simulink model "EXPERIMENT_03"  (R2023b)
settings: Solver=VariableStepAuto  StartTime=0.0  StopTime=0.2  RelTol=1e-3
libraries: spsRMSLib x24, spsPowerLib x16, spsVoltageMeasurementLib x16, spsSeriesRLCBranchLib x15, spsACVoltageSourceLib x8, spsCurrentMeasurementLib x8, spsSeriesRLCLoadLib x8, sps_lib x1
settings Model: Creator=deves  LastModifiedBy=deves

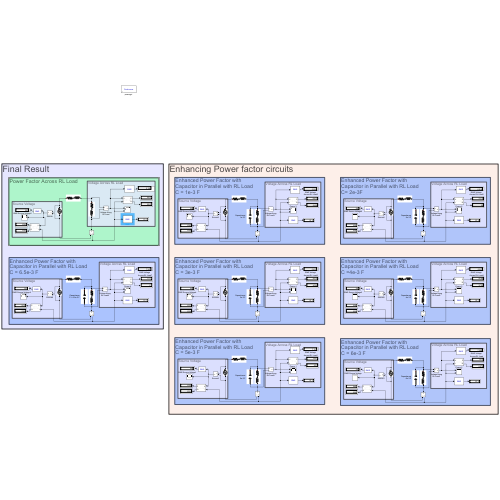
[thumbnail: Simulink's stored preview of the top-level diagram]
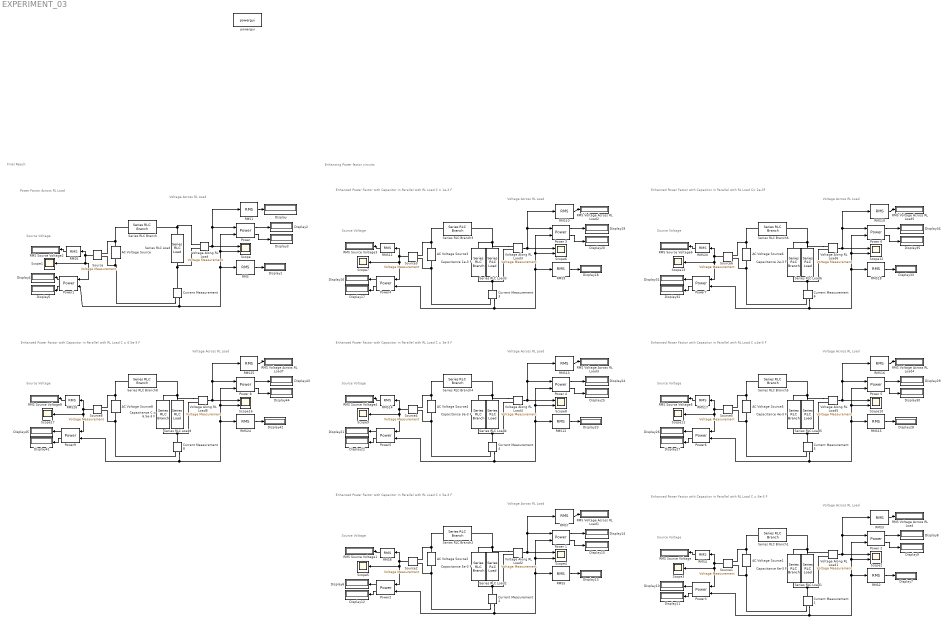
== system EXPERIMENT_03 ==
  note: Final Result
  note: Enhancing Power factor circuits
  note: Enhanced Power Factor with
      | Capacitor in Parallel with RL Load
      | C = 6e-3 F
  note: Power Factor Across RL Load
  note: Source Voltage
  note: Voltage Across RL Load
  note: Voltage Across RL Load
  note: Source Voltage
  note: Voltage Across RL Load
  note: Source Voltage
  note: Enhanced Power Factor with
      | Capacitor in Parallel with RL Load
      | C = 5e-3 F
  note: Voltage Across RL Load
  note: Source Voltage
  note: Enhanced Power Factor with
      | Capacitor in Parallel with RL Load
      | C = 1e-3 F
  note: Voltage Across RL Load
  note: Source Voltage
  note: Enhanced Power Factor with
      | Capacitor in Parallel with RL Load
      | C = 3e-3 F
  note: Voltage Across RL Load
  note: Source Voltage
  note: Enhanced Power Factor with
      | Capacitor in Parallel with RL Load
      | C =4e-3 F
  note: Voltage Across RL Load
  note: Source Voltage
  note: Enhanced Power Factor with
      | Capacitor in Parallel with RL Load
      | C= 2e-3F
  note: Enhanced Power Factor with
      | Capacitor in Parallel with RL Load
      | C = 6.5e-3 F
  note: Voltage Across RL Load
  note: Source Voltage
  AC Voltage Source{,1..6,8} (8 alike) : spsACVoltageSourceLib/AC Voltage Source  Amplitude=220*sqrt(2)  Phase=0  Frequency=50  SampleTime=.0001  Measurements=None  BusType=swing  Pref=10e3  Qref=0  Qmin=-inf  Qmax=+inf
  Capacitance 1e-3 F : spsSeriesRLCBranchLib/Series RLC Branch  LConnTagsString=__new0  RConnTagsString=__new0  BranchType=C  Resistance=1  Inductance=1e-3  SetiL0=off  InitialCurrent=0  Capacitance=1e-3  Setx0=off  InitialVoltage=0  Measurements=None
  Capacitance 2e-3 F : spsSeriesRLCBranchLib/Series RLC Branch  LConnTagsString=__new0  RConnTagsString=__new0  BranchType=C  Resistance=1  Inductance=1e-3  SetiL0=off  InitialCurrent=0  Capacitance=2e-3  Setx0=off  InitialVoltage=0  Measurements=None
  Capacitance 3e-3 F : spsSeriesRLCBranchLib/Series RLC Branch  LConnTagsString=__new0  RConnTagsString=__new0  BranchType=C  Resistance=1  Inductance=1e-3  SetiL0=off  InitialCurrent=0  Capacitance=3e-3  Setx0=off  InitialVoltage=0  Measurements=None
  Capacitance 4e-3 F : spsSeriesRLCBranchLib/Series RLC Branch  LConnTagsString=__new0  RConnTagsString=__new0  BranchType=C  Resistance=1  Inductance=1e-3  SetiL0=off  InitialCurrent=0  Capacitance=4e-3  Setx0=off  InitialVoltage=0  Measurements=None
  Capacitance 5e-3 F : spsSeriesRLCBranchLib/Series RLC Branch  LConnTagsString=__new0  RConnTagsString=__new0  BranchType=C  Resistance=1  Inductance=1e-3  SetiL0=off  InitialCurrent=0  Capacitance=5e-3  Setx0=off  InitialVoltage=0  Measurements=None
  Capacitance 6e-3 F : spsSeriesRLCBranchLib/Series RLC Branch  LConnTagsString=__new0  RConnTagsString=__new0  BranchType=C  Resistance=1  Inductance=1e-3  SetiL0=off  InitialCurrent=0  Capacitance=6e-3  Setx0=off  InitialVoltage=0  Measurements=None
  Capacitance C = 6.5e-3 F : spsSeriesRLCBranchLib/Series RLC Branch  LConnTagsString=__new0  RConnTagsString=__new0  BranchType=C  Resistance=1  Inductance=1e-3  SetiL0=off  InitialCurrent=0  Capacitance=6.5e-3  Setx0=off  InitialVoltage=0  Measurements=None
  Current Measurement{,1..6,8} (8 alike) : spsCurrentMeasurementLib/Current Measurement  PhasorSimulation=off  OutputType=Complex  PSBequivalent=0
  Display{,1..35,41..45} (41 alike) : Display
  Power{,1..7,9} (9 alike) : spsPowerLib/Power  Freq=50  Vinit=[1, 0]  Iinit=[1, 0]  Ts=0
  Power {1..6,8} (7 alike) : spsPowerLib/Power  Freq=50  Vinit=[1, 0]  Iinit=[1, 0]  Ts=0
  RMS{,1..20,24..26} (24 alike) : spsRMSLib/RMS  TrueRMS=on  Freq=50  RMSInit=120  Ts=0
  RMS Source Voltage{,1..6,8} (8 alike) : Display
  RMS Voltage Across RL Load{,1..5,7} (7 alike) : Display
  Scope{,2,4,6,8,10,12,16} (8 alike) : Scope  NumInputPorts=2
  Scope{1,3,5,7,9,11,13,17} (8 alike) : Scope
  Series RLC Branch{,1..6,8} (8 alike) : spsSeriesRLCBranchLib/Series RLC Branch  LConnTagsString=__new0  RConnTagsString=__new0  BranchType=RL  Resistance=10  Inductance=3.183e-2  SetiL0=off  InitialCurrent=0  Capacitance=1e-6  Setx0=off  InitialVoltage=0  Measurements=None
  Series RLC Load{,1..6,8} (8 alike) : spsSeriesRLCLoadLib/Series RLC Load  LConnTagsString=a  RConnTagsString=__new0  NominalVoltage=220  NominalFrequency=50  ActivePower=10e4  InductivePower=10e4  CapacitivePower=0  Setx0=off  InitialVoltage=0  SetiL0=off  InitialCurrent=0  Measurements=None  LoadType=constant Z
  Source{,1..6,8} (8 alike) : spsVoltageMeasurementLib/Voltage Measurement  PhasorSimulation=off  OutputType=Complex  PSBequivalent=0
  Voltage Along RL Load{,1..6,8} (8 alike) : spsVoltageMeasurementLib/Voltage Measurement  PhasorSimulation=off  OutputType=Complex  PSBequivalent=0
  powergui : sps_lib/powergui  Priority=1  SimulationMode=Continuous  SampleTime=50e-6  frequency=60  Iterations=50  frequencyindice=50  Pbase=100e6  ErrMax=1e-4  UnitsV=kV  UnitsW=MW  buscounter=0  FunctionMessages=off  echomessages=off  EnableUseOfTLC=off  CurrentSourceSwitches=off  DisableSnubberDevices=off  DisableRonSwitches=off  DisableVfSwitches=off  DisplayEquations=off  AutomaticDiscreteSolvers=off  SolverType=Tustin/Backward Euler (TBE)  Interpol=off  ExternalGateDelay=off  methode=off  Ts=100  x0status=blocks  SPID=on  SwTol=0  HookPort=off  NonlinearTolerance=1e-4  nMaxIteration=100  ContinueOnMaxIteration=off  RestoreLinks=warning  ResistiveCurrentMeasurement=off  Frange=[0:2:500]  Ylog=off  Xlog=on  ShowGrid=off  save=off  variable=ZData  structure=0  ZoomFFT=off  StartTime=0.0  cycles=1  DisplayStyle=1  fundamental=60  FreqAxis=off  MaxFrequency=1000  frequencyindicesteady=1  RmsSteady=1  display=off
  wires:
  Source/1 -> Scope1/1, Power1/1, RMS6/1
  Current Measurement/1 -> Scope/2, Power/2, RMS/1, Power1/2
  Voltage Along RL Load/1 -> RMS1/1, Power/1, Scope/1
  RMS1/1 -> Display/1
  RMS/1 -> Display1/1
  Power/1 -> Display2/1
  Power/2 -> Display3/1
  Power1/2 -> Display5/1
  Power1/1 -> Display4/1
  Power3/1 -> Display10/1
  RMS2/1 -> Display7/1
  Voltage Along RL Load1/1 -> RMS3/1, Power 2/1, Scope2/1
  RMS3/1 -> RMS Voltage Across RL Load/1
  Source1/1 -> Scope3/1, Power3/1, RMS4/1
  Power3/2 -> Display11/1
  Power 2/2 -> Display9/1
  Current Measurement1/1 -> Scope2/2, Power 2/2, RMS2/1, Power3/2
  Power 2/1 -> Display8/1
  RMS4/1 -> RMS Source Voltage/1
  RMS6/1 -> RMS Source Voltage2/1
  RMS7/1 -> RMS Voltage Across RL Load1/1
  RMS8/1 -> RMS Source Voltage1/1
  Power2/1 -> Display6/1
  Power 1/1 -> Display14/1
  Current Measurement2/1 -> Scope4/2, Power 1/2, RMS5/1, Power2/2
  Power 1/2 -> Display15/1
  Source2/1 -> Scope5/1, Power2/1, RMS8/1
  Voltage Along RL Load2/1 -> RMS7/1, Power 1/1, Scope4/1
  RMS5/1 -> Display13/1
  Power2/2 -> Display12/1
  RMS10/1 -> RMS Voltage Across RL Load2/1
  RMS11/1 -> RMS Source Voltage3/1
  Power4/1 -> Display16/1
  Power 3/1 -> Display19/1
  Current Measurement3/1 -> Scope6/2, Power 3/2, RMS9/1, Power4/2
  Power 3/2 -> Display20/1
  Source3/1 -> Scope7/1, Power4/1, RMS11/1
  Voltage Along RL Load3/1 -> RMS10/1, Power 3/1, Scope6/1
  RMS9/1 -> Display18/1
  Power4/2 -> Display17/1
  RMS13/1 -> RMS Voltage Across RL Load3/1
  RMS14/1 -> RMS Source Voltage4/1
  Power5/1 -> Display21/1
  Power 4/1 -> Display24/1
  Current Measurement4/1 -> Scope8/2, Power 4/2, RMS12/1, Power5/2
  Power 4/2 -> Display25/1
  Source4/1 -> Scope9/1, Power5/1, RMS14/1
  Voltage Along RL Load4/1 -> RMS13/1, Power 4/1, Scope8/1
  RMS12/1 -> Display23/1
  Power5/2 -> Display22/1
  RMS16/1 -> RMS Voltage Across RL Load4/1
  RMS17/1 -> RMS Source Voltage5/1
  Power6/1 -> Display26/1
  Power 5/1 -> Display29/1
  Current Measurement5/1 -> Scope10/2, Power 5/2, RMS15/1, Power6/2
  Power 5/2 -> Display30/1
  Source5/1 -> Scope11/1, Power6/1, RMS17/1
  Voltage Along RL Load5/1 -> RMS16/1, Power 5/1, Scope10/1
  RMS15/1 -> Display28/1
  Power6/2 -> Display27/1
  RMS19/1 -> RMS Voltage Across RL Load5/1
  RMS20/1 -> RMS Source Voltage6/1
  Power7/1 -> Display31/1
  Power 6/1 -> Display34/1
  Current Measurement6/1 -> Scope12/2, Power 6/2, RMS18/1, Power7/2
  Power 6/2 -> Display35/1
  Source6/1 -> Scope13/1, Power7/1, RMS20/1
  Voltage Along RL Load6/1 -> RMS19/1, Power 6/1, Scope12/1
  RMS18/1 -> Display33/1
  Power7/2 -> Display32/1
  Power9/2 -> Display41/1
  Source8/1 -> Scope17/1, Power9/1, RMS26/1
  Voltage Along RL Load8/1 -> RMS25/1, Power 8/1, Scope16/1
  RMS24/1 -> Display42/1
  RMS26/1 -> RMS Source Voltage8/1
  RMS25/1 -> RMS Voltage Across RL Load7/1
  Power 8/1 -> Display43/1
  Power9/1 -> Display45/1
  Current Measurement8/1 -> Scope16/2, Power 8/2, RMS24/1, Power9/2
  Power 8/2 -> Display44/1
  connections:
  Source/LConn1 -- Series RLC Branch/LConn1 -- AC Voltage Source/RConn1
  Current Measurement/RConn1 -- AC Voltage Source/LConn1 -- Source/LConn2
  Series RLC Load/LConn1 -- Voltage Along RL Load/LConn1 -- Series RLC Branch/RConn1
  Current Measurement/LConn1 -- Voltage Along RL Load/LConn2 -- Series RLC Load/RConn1
  Series RLC Load1/LConn1 -- Capacitance 6e-3 F/LConn1 -- Series RLC Branch1/RConn1 -- Voltage Along RL Load1/LConn1
  AC Voltage Source1/RConn1 -- Series RLC Branch1/LConn1 -- Source1/LConn1
  Source1/LConn2 -- Current Measurement1/RConn1 -- AC Voltage Source1/LConn1
  Current Measurement1/LConn1 -- Capacitance 6e-3 F/RConn1 -- Voltage Along RL Load1/LConn2 -- Series RLC Load1/RConn1
  Series RLC Load2/RConn1 -- Current Measurement2/LConn1 -- Capacitance 5e-3 F/RConn1 -- Voltage Along RL Load2/LConn2
  AC Voltage Source2/LConn1 -- Current Measurement2/RConn1 -- Source2/LConn2
  Source2/LConn1 -- Series RLC Branch2/LConn1 -- AC Voltage Source2/RConn1
  Voltage Along RL Load2/LConn1 -- Series RLC Load2/LConn1 -- Capacitance 5e-3 F/LConn1 -- Series RLC Branch2/RConn1
  Series RLC Load3/RConn1 -- Current Measurement3/LConn1 -- Capacitance 1e-3 F/RConn1 -- Voltage Along RL Load3/LConn2
  AC Voltage Source3/LConn1 -- Current Measurement3/RConn1 -- Source3/LConn2
  Source3/LConn1 -- Series RLC Branch3/LConn1 -- AC Voltage Source3/RConn1
  Voltage Along RL Load3/LConn1 -- Series RLC Load3/LConn1 -- Capacitance 1e-3 F/LConn1 -- Series RLC Branch3/RConn1
  Series RLC Load4/RConn1 -- Current Measurement4/LConn1 -- Capacitance 3e-3 F/RConn1 -- Voltage Along RL Load4/LConn2
  AC Voltage Source4/LConn1 -- Current Measurement4/RConn1 -- Source4/LConn2
  Source4/LConn1 -- Series RLC Branch4/LConn1 -- AC Voltage Source4/RConn1
  Voltage Along RL Load4/LConn1 -- Series RLC Load4/LConn1 -- Capacitance 3e-3 F/LConn1 -- Series RLC Branch4/RConn1
  Series RLC Load5/RConn1 -- Current Measurement5/LConn1 -- Capacitance 4e-3 F/RConn1 -- Voltage Along RL Load5/LConn2
  AC Voltage Source5/LConn1 -- Current Measurement5/RConn1 -- Source5/LConn2
  Source5/LConn1 -- Series RLC Branch5/LConn1 -- AC Voltage Source5/RConn1
  Voltage Along RL Load5/LConn1 -- Series RLC Load5/LConn1 -- Capacitance 4e-3 F/LConn1 -- Series RLC Branch5/RConn1
  Series RLC Load6/RConn1 -- Current Measurement6/LConn1 -- Capacitance 2e-3 F/RConn1 -- Voltage Along RL Load6/LConn2
  AC Voltage Source6/LConn1 -- Current Measurement6/RConn1 -- Source6/LConn2
  Source6/LConn1 -- Series RLC Branch6/LConn1 -- AC Voltage Source6/RConn1
  Voltage Along RL Load6/LConn1 -- Series RLC Load6/LConn1 -- Capacitance 2e-3 F/LConn1 -- Series RLC Branch6/RConn1
  Voltage Along RL Load8/LConn1 -- Series RLC Load8/LConn1 -- Capacitance C = 6.5e-3 F/LConn1 -- Series RLC Branch8/RConn1
  AC Voltage Source8/LConn1 -- Current Measurement8/RConn1 -- Source8/LConn2
  AC Voltage Source8/RConn1 -- Series RLC Branch8/LConn1 -- Source8/LConn1
  Series RLC Load8/RConn1 -- Current Measurement8/LConn1 -- Capacitance C = 6.5e-3 F/RConn1 -- Voltage Along RL Load8/LConn2
